simulink subsystem "Subsystem_Encoder_ACT"  (R2023b)
settings: Solver=VariableStepAuto  StartTime=0.0  StopTime=10.0  RelTol=1e-3
libraries: arduinosensorlib x2
settings Model: Creator=Alberto  LastModifiedBy=Gonzalo

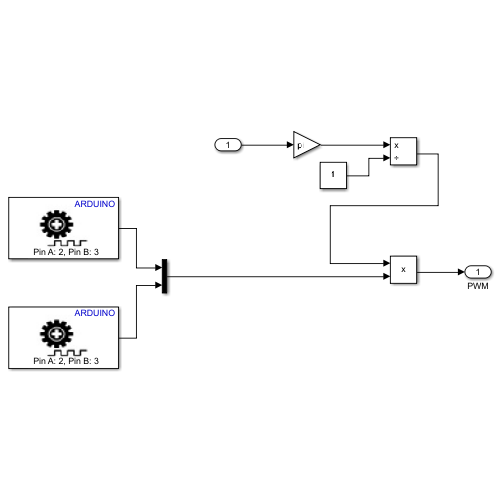
[thumbnail: Simulink's stored preview of the top-level diagram]
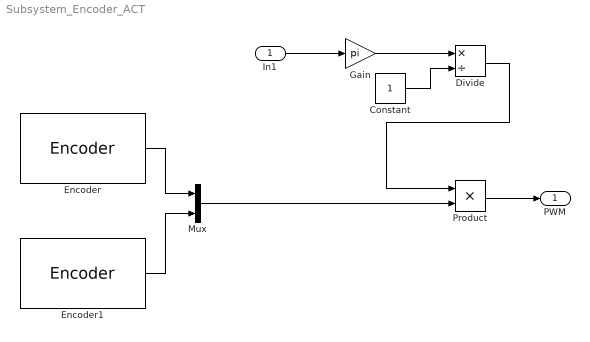
== system Subsystem_Encoder_ACT ==
  In1 : Inport
  Constant : Constant
  Divide : Product  Inputs=*/
  Encoder : arduinosensorlib/Encoder  InputA=2  InputB=3  Mode=No reset  SampleTime=-1
  Encoder1 : arduinosensorlib/Encoder  InputA=2  InputB=3  Mode=No reset  SampleTime=-1
  Gain : Gain  Gain=pi
  Mux : Mux  Inputs=2
  Product : Product
  PWM : Outport
  wires:
  Encoder/1 -> Mux/1
  Encoder1/1 -> Mux/2
  Mux/1 -> Product/2
  In1/1 -> Gain/1
  Gain/1 -> Divide/1
  Constant/1 -> Divide/2
  Divide/1 -> Product/1
  Product/1 -> PWM/1
